simulink library "AEMS_Standard_Library"  (R2016b)
settings: Solver=ode45  StartTime=0.0  StopTime=10.0  RelTol=1e-3
undefined symbols (not defined in the file or in its folder): BkPY, carto, Cbx_extegr, Cbx_lpegrsys, Cbx_portegr, Cnx_bnk_nr_conf, Cnx_cyl_nr_conf, ConfigManagement, configuration_management, Cxx_dcm_io_tmr_end_xxxx, Cxx_dcm_rt_tmr_end, Cxx_DID_xxxx_IO_max, Cxx_DID_xxxx_IO_min, Cxx_egrhsofs, Cxx_vmaniegi, DEM_DEBOUNCE_FREEZE, DEM_DTR_CTL_INVISIBLE, DEM_DTR_CTL_NORMAL, Dem_DtrId2_XXX, Dem_DtrId3_XXX, Dem_DtrId4_XXX, Dem_DtrId5_XXX, Dem_DtrId6_XXX, Dem_DtrId7_XXX, Dem_DtrId8_XXX, Dem_DtrId9_XXX, Dem_DtrId_XXX, Dem_EnableConditionId2_XXX, Dem_EnableConditionId3_XXX, Dem_EnableConditionId4_XXX, Dem_EnableConditionId5_XXX, Dem_EnableConditionId6_XXX, Dem_EnableConditionId7_XXX, Dem_EnableConditionId8_XXX, Dem_EnableConditionId_XXX, Dem_EventId, Dem_EventId2_XXX, Dem_EventId3_XXX, Dem_EventId4_XXX, Dem_EventId5_XXX, Dem_EventId6_XXX, Dem_EventId7_XXX, Dem_EventId8_XXX, Dem_EventId9_XXX, Dem_EventId_Device_Faulttype, Dem_EventId_XXX, DEM_IUMPR_GENERAL_DENOMINATOR, DEM_OPCYC_IGNITION, Dem_RatioId2_XXX, Dem_RatioId3_XXX, Dem_RatioId4_XXX, Dem_RatioId5_XXX, Dem_RatioId6_XXX, Dem_RatioId7_XXX, Dem_RatioId8_XXX, Dem_RatioId_XXX, Dem_StorageConditionId2_XXX, Dem_StorageConditionId3_XXX, Dem_StorageConditionId4_XXX, Dem_StorageConditionId5_XXX ... (+65)
libraries: AEMS_Standard_Library x477, simulink x2
(part 36 of 39)

== system AEMS_Standard_Library/SUB/AEMS_SORT_MEDIAN/Pair ==
  Vector_size : Inport
  Sorted_vector : Inport  Port=2
  Action Port : ActionPort
  Add : Sum  OutDataTypeStr=Inherit: Inherit via back propagation
  Add1 : Sum  OutDataTypeStr=Inherit: Inherit via back propagation  SaturateOnIntegerOverflow=on  InputSameDT=on
  Constant : Constant  Value=2  OutDataTypeStr=uint8
  Constant1 : Constant  OutDataTypeStr=uint8
  Constant2 : Constant  Value=2  OutDataTypeStr=uint8
  Divide : Product  Inputs=*/  OutDataTypeStr=Inherit: Inherit via back propagation
  Divide1 : Product  Inputs=*/  OutDataTypeStr=Inherit: Inherit via back propagation
  Selector : Selector  IndexMode=Zero-based  InputPortWidth=N  IndexOptions=Index vector (port)  Indices=[1 3]  OutputSizes=1
  Selector1 : Selector  IndexMode=Zero-based  InputPortWidth=N  IndexOptions=Index vector (port)  Indices=[1 3]  OutputSizes=1
  Median_Pair : Outport
  wires:
  Constant/1 -> Divide/2
  Divide/1 -> Selector/2, Add/1
  Constant1/1 -> Add/2
  Add/1 -> Selector1/2
  Selector/1 -> Add1/1
  Selector1/1 -> Add1/2
  Add1/1 -> Divide1/1
  Constant2/1 -> Divide1/2
  Divide1/1 -> Median_Pair/1
  Vector_size/1 -> Divide/1
  Sorted_vector/1 -> Selector1/1, Selector/1

== system AEMS_Standard_Library/TIMER/AEMS_TIMER1/EdgeRising ==
  In : Inport
  DelayInput1 : UnitDelay  Description=\nStore in Global RAM  InitialCondition=initinit  SampleTime=-1
      settings: AttributesFormatString=IC = %<X0>
  LogicalOperator1 : Logic  OutDataTypeStr=boolean
  LogicalOperator3 : Logic  Operator=NOT  Inputs=1  OutDataTypeStr=boolean
  Out : Outport
  wires:
  LogicalOperator1/1 -> Out/1
  In/1 -> LogicalOperator1/1, DelayInput1/1
  DelayInput1/1 -> LogicalOperator3/1
  LogicalOperator3/1 -> LogicalOperator1/2

== system AEMS_Standard_Library/COM/AEMS_FRAME_SUPERVISION/ecu_frm_detection/C_mngt ==
  Frm_Detection_Cnd : Inport
  Status_Loc2 : Inport  Port=2
  Frm_Conf : Inport  Port=3
  Clear_Diag_Info_Counter : Inport  Port=4
  Frm_Detected_PREV : Inport  Port=5
  Constant10 : Constant  Value=0  OutDataTypeStr=Inherit: Inherit via back propagation
  Constant2 : Constant  OutDataTypeStr=Inherit: Inherit via back propagation
  Constant3 : Constant  Value=false
  Constant8 : Constant  Value=Nnx_pres_stt
  DataTypeConversion1 : DataTypeConversion  RndMeth=Zero
  LogicalOperator2 : Logic  Inputs=3  OutDataTypeStr=boolean
  LogicalOperator3 : Logic  Operator=OR  Inputs=3  OutDataTypeStr=boolean
  RelationalOperator1 : RelationalOperator  Operator===  OutDataTypeStr=boolean  RndMeth=Nearest  InputSameDT=on
  RelationalOperator2 : RelationalOperator  Operator===  OutDataTypeStr=boolean  RndMeth=Nearest  InputSameDT=on
  RelationalOperator7 : RelationalOperator  Operator===  OutDataTypeStr=boolean  RndMeth=Nearest  InputSameDT=on
  Switch : Switch  Criteria=u2 ~= 0
      settings: AttributesFormatString=Criteria=%<Criteria>
  Frm_Detected : Outport
  wires:
  Switch/1 -> DataTypeConversion1/1
  Clear_Diag_Info_Counter/1 -> Switch/2
  Constant10/1 -> RelationalOperator2/2
  RelationalOperator7/1 -> LogicalOperator2/3
  Constant8/1 -> RelationalOperator7/1
  Frm_Detection_Cnd/1 -> LogicalOperator2/2
  RelationalOperator2/1 -> LogicalOperator3/1
  LogicalOperator2/1 -> LogicalOperator3/2
  Frm_Conf/1 -> RelationalOperator2/1, RelationalOperator1/1
  RelationalOperator1/1 -> LogicalOperator2/1
  Constant2/1 -> RelationalOperator1/2
  Frm_Detected_PREV/1 -> LogicalOperator3/3
  LogicalOperator3/1 -> Switch/1
  DataTypeConversion1/1 -> Frm_Detected/1
  Status_Loc2/1 -> RelationalOperator7/2
  Constant3/1 -> Switch/3

== system AEMS_Standard_Library/COM/AEMS_FRAME_SUPERVISION/ecu_frm_monitoring/A_Monitoring_Condition ==
  GADE : Inport
  ECU_Category : Inport  Port=2
  IgnitionSupplyConfirmation : Inport  Port=3
  Specific_Mon_Cnd : Inport  Port=4
  Frame_Detected_Loc2 : Inport  Port=5
  BCM_Status : Inport  Port=6
  USM_Status : Inport  Port=7
  GADEOK : Constant  Value=3  OutDataTypeStr=Inherit: Inherit via back propagation
  LogicalOperator1 : Logic  OutDataTypeStr=boolean
  LogicalOperator2 : Logic  Inputs=3  OutDataTypeStr=boolean
  LogicalOperator3 : Logic  Operator=OR  OutDataTypeStr=boolean
  PRESENTSTATUS : Constant  Value=Nnx_pres_stt
  PRESENTSTATUS_102 : Constant  Value=Nnx_pres_stt
  RelationalOperator1 : RelationalOperator  Operator===  OutDataTypeStr=boolean  RndMeth=Nearest  InputSameDT=on
  RelationalOperator2 : RelationalOperator  Operator=~=  OutDataTypeStr=boolean  RndMeth=Nearest  InputSameDT=on
  RelationalOperator3 : RelationalOperator  Operator===  OutDataTypeStr=boolean  RndMeth=Nearest  InputSameDT=on
  Switch : Switch  Criteria=u2 ~= 0  RndMeth=Zero  InputSameDT=on
      settings: AttributesFormatString=Criteria=%<Criteria>
  Mon_Authorize : Outport
  wires:
  LogicalOperator3/1 -> Switch/1
  LogicalOperator1/1 -> Switch/3
  LogicalOperator2/1 -> Mon_Authorize/1
  BCM_Status/1 -> RelationalOperator1/1
  Frame_Detected_Loc2/1 -> LogicalOperator2/3
  Specific_Mon_Cnd/1 -> LogicalOperator2/2
  Switch/1 -> LogicalOperator2/1
  PRESENTSTATUS_102/1 -> RelationalOperator2/2
  USM_Status/1 -> RelationalOperator2/1
  PRESENTSTATUS/1 -> RelationalOperator1/2
  RelationalOperator2/1 -> LogicalOperator3/2
  IgnitionSupplyConfirmation/1 -> LogicalOperator3/1
  RelationalOperator1/1 -> LogicalOperator1/1
  RelationalOperator3/1 -> LogicalOperator1/2
  GADEOK/1 -> RelationalOperator3/2
  GADE/1 -> RelationalOperator3/1
  ECU_Category/1 -> Switch/2

== system AEMS_Standard_Library/COM/AEMS_FRAME_SUPERVISION/ecu_frm_monitoring/B_Status_Management ==
  rcpt_frm : Inport
  Mon_Authorize : Inport  Port=2
  TimeSched_dt : Inport  Port=3
  JT1 : Inport  Port=4
  JT2 : Inport  Port=5
  Vbx_atsr_sys_ecu_ini_task10ms : Inport  Port=6
  Frame_Detected : Inport  Port=7
  C_Status_building : Subsystem
  Constant : Constant  Value=Nnx_pres_stt
  Constant1 : Constant  Value=Nnx_abst_stt
  Switch : Switch  Criteria=u2 ~= 0
      settings: AttributesFormatString=Criteria=%<Criteria>
  Switch3 : Switch  Criteria=u2 ~= 0  RndMeth=Zero  InputSameDT=on
      settings: AttributesFormatString=Criteria=%<Criteria>
  Unit Delay : UnitDelay  SampleTime=-1
      settings: AttributesFormatString=<initial=%<InitialCondition>>
  Status : Outport
  wires:
  Unit Delay/1 -> C_Status_building/6(Status_PREV)
  Switch/1 -> Status/1, Unit Delay/1
  rcpt_frm/1 -> C_Status_building/5(Frame_Received)
  Frame_Detected/1 -> Switch3/2
  Constant/1 -> Switch3/1
  Constant1/1 -> Switch3/3
  Vbx_atsr_sys_ecu_ini_task10ms/1 -> Switch/2
  Mon_Authorize/1 -> C_Status_building/1(Mon_Authorize)
  TimeSched_dt/1 -> C_Status_building/2(TimeSched_dt)
  JT1/1 -> C_Status_building/3(JT1)
  JT2/1 -> C_Status_building/4(JT2)
  Switch3/1 -> Switch/1
  C_Status_building/1(Status) -> Switch/3

== system AEMS_Standard_Library/COM/AEMS_FRAME_SUPERVISION/ecu_monitoring_display/D_ctr_mem_max ==
  VALMAX : Inport
  M_Absent_PREV : Inport  Port=2
  Vbx_rcpt_XXX_mon_PREV : Inport  Port=3
  IGN_Status : Inport  Port=4
  decM : Inport  Port=5
  decThres : Inport  Port=6
  Frame_Received_Counter : Inport  Port=7
  Clear_Diag_Info_Counter : Inport  Port=8
  Status : Inport  Port=9
  Constant : Constant  Value=Nnx_vld_abst_stt
  Constant1 : Constant  Value=0  OutDataTypeStr=Inherit: Inherit via back propagation
  Constant2 : Constant  Value=0  OutDataTypeStr=Inherit: Inherit via back propagation
  DataTypeConversion2 : DataTypeConversion  RndMeth=Zero
  LogicalOperator : Logic  Operator=NOT  OutDataTypeStr=boolean
  LogicalOperator1 : Logic  Operator=OR  OutDataTypeStr=boolean
  LogicalOperator2 : Logic  Operator=OR  OutDataTypeStr=boolean
  LogicalOperator3 : Logic  Inputs=3  OutDataTypeStr=boolean
  MinMax : MinMax  Function=max  Inputs=2  OutDataTypeStr=Inherit: Inherit via back propagation  RndMeth=Zero  InputSameDT=on
  RelationalOperator2 : RelationalOperator  Operator=~=  OutDataTypeStr=boolean  RndMeth=Nearest  InputSameDT=on
  RelationalOperator4 : RelationalOperator  Operator===  OutDataTypeStr=boolean  RndMeth=Nearest  InputSameDT=on
  RelationalOperator5 : RelationalOperator  Operator=<  OutDataTypeStr=boolean  RndMeth=Nearest  InputSameDT=on
  Subtract : Sum  Inputs=+-  OutDataTypeStr=Inherit: Inherit via back propagation  RndMeth=Zero  InputSameDT=on
  Switch{1..6} (6 alike) : Switch  Criteria=u2 ~= 0  RndMeth=Zero  SaturateOnIntegerOverflow=on  InputSameDT=on
      settings: AttributesFormatString=Criteria=%<Criteria>
  M_Absent : Outport
  Vbx_rcpt_XXX_mon : Outport  Port=2
  wires:
  Frame_Received_Counter/1 -> Switch5/2, Switch6/2
  Constant/1 -> RelationalOperator4/2
  Status/1 -> RelationalOperator4/1
  VALMAX/1 -> Switch1/1
  RelationalOperator4/1 -> LogicalOperator1/1, Switch1/2
  Switch6/1 -> Vbx_rcpt_XXX_mon/1
  LogicalOperator1/1 -> Switch6/1
  LogicalOperator2/1 -> Switch6/3
  Switch1/1 -> Switch5/1
  LogicalOperator3/1 -> Switch4/2
  Vbx_rcpt_XXX_mon_PREV/1 -> LogicalOperator1/2, LogicalOperator/1, LogicalOperator2/1
  Constant1/1 -> RelationalOperator2/2
  M_Absent_PREV/1 -> Subtract/1, Switch4/3, RelationalOperator2/1, Switch2/3, RelationalOperator5/2, Switch1/3
  RelationalOperator2/1 -> LogicalOperator3/3
  IGN_Status/1 -> LogicalOperator2/2, LogicalOperator3/2
  LogicalOperator/1 -> LogicalOperator3/1
  Switch4/1 -> Switch5/3
  Switch5/1 -> Switch3/1
  Switch3/1 -> DataTypeConversion2/1
  Clear_Diag_Info_Counter/1 -> Switch3/2
  Constant2/1 -> Switch3/3
  DataTypeConversion2/1 -> M_Absent/1
  RelationalOperator5/1 -> Switch2/2
  decM/1 -> Switch2/1, RelationalOperator5/1
  Switch2/1 -> Subtract/2
  Subtract/1 -> MinMax/1
  decThres/1 -> MinMax/2
  MinMax/1 -> Switch4/1

== system AEMS_Standard_Library/COM/AEMS_FRAME_SUPERVISION/ecu_monitoring_display/E_diag_display ==
  note: b1000 0000
  note: b1100 0000
  note: b1111 1111
  note: b0011 1111
  M_Absent : Inport
  Mon_Authorized : Inport  Port=2
  Dspl_Mask_Cnd : Inport  Port=3
  Status : Inport  Port=4
  Constant : Constant  Value=Nnx_vld_abst_stt
  Constant1 : Constant  Value=Nnx_abst_stt
  Constant10 : Constant  Value=0  OutDataTypeStr=Inherit: Inherit via back propagation
  Constant2 : Constant  Value=63  OutDataTypeStr=Inherit: Inherit via back propagation
  Constant6 : Constant  Value=255  OutDataTypeStr=Inherit: Inherit via back propagation
  Constant7 : Constant  Value=128  OutDataTypeStr=Inherit: Inherit via back propagation
  Constant8 : Constant  Value=0  OutDataTypeStr=Inherit: Inherit via back propagation
  Constant9 : Constant  Value=192  OutDataTypeStr=Inherit: Inherit via back propagation
  LogicalOperator1 : Logic  Operator=NOT  Inputs=1  OutDataTypeStr=boolean
  LogicalOperator8 : Logic  Operator=OR  OutDataTypeStr=boolean
  MinMax : MinMax  Inputs=2  OutDataTypeStr=Inherit: Inherit via back propagation  RndMeth=Zero  InputSameDT=on
  RelationalOperator3 : RelationalOperator  Operator===  OutDataTypeStr=boolean  RndMeth=Nearest  InputSameDT=on
  RelationalOperator4 : RelationalOperator  Operator===  OutDataTypeStr=boolean  RndMeth=Nearest  InputSameDT=on
  Sum : Sum  Inputs=2  OutDataTypeStr=Inherit: Inherit via back propagation  RndMeth=Zero  InputSameDT=on
  Sum1 : Sum  Inputs=2  OutDataTypeStr=Inherit: Inherit via back propagation  RndMeth=Zero  InputSameDT=on
  Switch1 : Switch  Criteria=u2 ~= 0  RndMeth=Zero  SaturateOnIntegerOverflow=on  InputSameDT=on
      settings: AttributesFormatString=Criteria=%<Criteria>
  Switch2 : Switch  Criteria=u2 ~= 0  RndMeth=Zero  SaturateOnIntegerOverflow=on  InputSameDT=on
      settings: AttributesFormatString=Criteria=%<Criteria>
  Switch3 : Switch  Criteria=u2 ~= 0  RndMeth=Zero  SaturateOnIntegerOverflow=on  InputSameDT=on
      settings: AttributesFormatString=Criteria=%<Criteria>
  Diagnosis_Byte : Outport
  wires:
  LogicalOperator8/1 -> Switch1/2
  Constant6/1 -> Switch1/1
  Status/1 -> RelationalOperator3/1, RelationalOperator4/2
  Constant/1 -> RelationalOperator3/2
  Constant1/1 -> RelationalOperator4/1
  RelationalOperator4/1 -> Switch2/2
  Constant7/1 -> Switch2/1
  Constant8/1 -> Switch2/3
  RelationalOperator3/1 -> Switch3/2
  Constant9/1 -> Switch3/1
  Constant10/1 -> Switch3/3
  Switch1/1 -> Diagnosis_Byte/1
  Mon_Authorized/1 -> LogicalOperator1/1
  LogicalOperator1/1 -> LogicalOperator8/1
  Dspl_Mask_Cnd/1 -> LogicalOperator8/2
  M_Absent/1 -> MinMax/1
  Constant2/1 -> MinMax/2
  Sum1/1 -> Switch1/3
  MinMax/1 -> Sum/1
  Switch2/1 -> Sum/2
  Switch3/1 -> Sum1/2
  Sum/1 -> Sum1/1

== system AEMS_Standard_Library/DCM/AEMS_DCM_CLEARDIAGNOSTICINFORMATION/Callback_Subsystem/Enable_Clear_Request_Subsystem ==
  Enable : EnablePort
  Logical Operator3 : Logic  Operator=NOT  OutDataTypeStr=boolean
  Unit Delay1 : UnitDelay  SampleTime=-1
      settings: AttributesFormatString=<initial=%<InitialCondition>>
  flag_clr_req : Outport  InitialOutput=0
      settings: AttributesFormatString=<initial=%<InitialOutput>>\n<whendisabled=%<OutputWhenDisabled>>
  wires:
  Unit Delay1/1 -> Logical Operator3/1
  Logical Operator3/1 -> flag_clr_req/1, Unit Delay1/1

== system AEMS_Standard_Library/DISCONTINUITIES/AEMS_MULTI_PORT_TIME_SWITCH/slop_on/SR_FlipFlop1 ==
  S : Inport
  R : Inport  Port=2
  Constant1 : Constant  Value=false
  Constant2 : Constant  Value=true
  Constant3 : Constant  Value=true
  Constant5 : Constant  Value=false
  Logical_Operator : Logic  OutDataTypeStr=boolean
  Logical_Operator3 : Logic  Operator=NOT  OutDataTypeStr=boolean
  Relational_Operator : RelationalOperator  Operator===  OutDataTypeStr=boolean  RndMeth=Nearest  InputSameDT=on
  Switch{,1..3} (4 alike) : Switch  Criteria=u2 ~= 0  RndMeth=Zero  InputSameDT=on
      settings: AttributesFormatString=Criteria=%<Criteria>
  Unit_Delay : UnitDelay  SampleTime=-1
      settings: AttributesFormatString=IC = %<X0>
  Q : Outport
  QNot : Outport  Port=2
  wires:
  Logical_Operator3/1 -> QNot/1
  S/1 -> Switch/2, Logical_Operator/2
  R/1 -> Switch1/2, Logical_Operator/1
  Constant3/1 -> Switch/1
  Switch1/1 -> Switch/3
  Constant5/1 -> Switch1/1
  Unit_Delay/1 -> Relational_Operator/1, Switch1/3
  Switch3/1 -> Logical_Operator3/1, Q/1, Unit_Delay/1
  Logical_Operator/1 -> Switch3/2, Relational_Operator/2
  Relational_Operator/1 -> Switch2/2
  Constant2/1 -> Switch2/1
  Constant1/1 -> Switch2/3
  Switch2/1 -> Switch3/1
  Switch/1 -> Switch3/3

== system AEMS_Standard_Library/DISCONTINUITIES/AEMS_MULTI_PORT_TIME_SWITCH/transient_timer/AEMS_DIVISION_BY_ZERO ==
  den : Inport  Tag=AM,In,0,1,Name,C;CMP,Port,PortWidth,SampleTime;
  num : Inport  Tag=AM,In,0,1,Name,C;CMP,Port,PortWidth,SampleTime;  Port=2
  ans_of_0div : Inport  Tag=AM,In,0,1,Name,C;CMP,Port,PortWidth,SampleTime;  Port=3
  Divide : Product  Inputs=*/  OutDataTypeStr=Inherit: Inherit via back propagation  RndMeth=Zero
  MinMax1 : MinMax  Function=max  Inputs=2  OutDataTypeStr=Inherit: Inherit via back propagation  RndMeth=Zero  InputSameDT=on
  RelationalOperator : RelationalOperator  Tag=AM,Std,2,1;CMP,Operator;  Operator=~=  OutDataTypeStr=boolean  RndMeth=Nearest  InputSameDT=on
  Switch2 : Switch  Tag=GEN,Threshold;AM,Switch,2,1;CMP,Threshold;  Criteria=u2 ~= 0  RndMeth=Zero  SaturateOnIntegerOverflow=on  InputSameDT=on
      settings: AttributesFormatString=Criteria=%<Criteria>
  imm_zero : Constant  Tag=AM,Constant,0,1,Value;CMP,Value;  Value=0  OutDataTypeStr=Inherit: Inherit via back propagation
  imm_zero3 : Constant  Tag=AM,Constant,0,1,Value;CMP,Value;  Value=0.064/2^53  OutDataTypeStr=Inherit: Inherit via back propagation
  ans : Outport  Tag=AM,Out,1,0,Name,NC;CMP,Port,OutputWhenDisabled,InitialOutput;
  wires:
  den/1 -> RelationalOperator/1, MinMax1/1
  imm_zero/1 -> RelationalOperator/2
  num/1 -> Divide/1
  imm_zero3/1 -> MinMax1/2
  RelationalOperator/1 -> Switch2/2
  ans_of_0div/1 -> Switch2/3
  MinMax1/1 -> Divide/2
  Divide/1 -> Switch2/1
  Switch2/1 -> ans/1

== system AEMS_Standard_Library/DISCONTINUITIES/AEMS_SLEW_RATE/Slew_rate/Slewing ==
  OUTPUT_Prev : Inport
  MAX_SLEW_RATE : Inport  Port=2
  MIN_SLEW_RATE : Inport  Port=3
  INPUT : Inport  Port=4
  RelationalOperator : RelationalOperator  Operator=<=  OutDataTypeStr=boolean  RndMeth=Nearest  InputSameDT=on
  RelationalOperator1 : RelationalOperator  OutDataTypeStr=boolean  RndMeth=Nearest  InputSameDT=on
  Sum : Sum  Inputs=+-  OutDataTypeStr=Inherit: Inherit via back propagation  RndMeth=Zero  InputSameDT=on
  Sum1 : Sum  OutDataTypeStr=Inherit: Inherit via back propagation  RndMeth=Zero  InputSameDT=on
  Switch : Switch  Criteria=u2 ~= 0  RndMeth=Zero  SaturateOnIntegerOverflow=on  InputSameDT=on
      settings: AttributesFormatString=Criteria=%<Criteria>
  Switch1 : Switch  Criteria=u2 ~= 0  RndMeth=Zero  SaturateOnIntegerOverflow=on  InputSameDT=on
      settings: AttributesFormatString=Criteria=%<Criteria>
  OUTPUT : Outport  InitialOutput=0
  wires:
  Sum1/1 -> OUTPUT/1
  INPUT/1 -> Sum/1
  MIN_SLEW_RATE/1 -> RelationalOperator1/2, Switch1/3
  Switch/1 -> Sum1/2
  OUTPUT_Prev/1 -> Sum1/1, Sum/2
  RelationalOperator/1 -> Switch/2
  Sum/1 -> RelationalOperator/2, RelationalOperator1/1, Switch1/1
  RelationalOperator1/1 -> Switch1/2
  Switch1/1 -> Switch/3
  MAX_SLEW_RATE/1 -> RelationalOperator/1, Switch/1

== system AEMS_Standard_Library/DISCONTINUITIES/AEMS_SLOPE_SWITCH/Slope_On_Block/Error_Due_To_High_Slope_Test ==
  Signal_Change : Inport
  Output_Less_Than_Input : Inport  Port=2
  Output_Greater_Than_Input : Inport  Port=3
  Logical_Operator1 : Logic  Operator=OR  OutDataTypeStr=boolean
  Relational_Operator3 : RelationalOperator  Operator=~=  OutDataTypeStr=boolean  RndMeth=Nearest  InputSameDT=on
  Unit_Delay1 : UnitDelay  SampleTime=-1
      settings: AttributesFormatString=IC = %<X0>
  Test_passed : Outport
  wires:
  Logical_Operator1/1 -> Test_passed/1
  Signal_Change/1 -> Logical_Operator1/1
  Output_Less_Than_Input/1 -> Unit_Delay1/1
  Output_Greater_Than_Input/1 -> Relational_Operator3/1
  Relational_Operator3/1 -> Logical_Operator1/2
  Unit_Delay1/1 -> Relational_Operator3/2

== system AEMS_Standard_Library/DISCONTINUITIES/AEMS_SLOPE_SWITCH/Slope_On_Block/Output_Comparision ==
  Test_passed : Inport
  Input : Inport  Tag=AM,In,0,1,Name,C;CMP,Port,PortWidth,SampleTime;  Port=2
  Pos_Slope : Inport  Tag=AM,In,0,1,Name,C;CMP,Port,PortWidth,SampleTime;  Port=3
  Prev_Output : Inport  Port=4
  Neg_Slope : Inport  Tag=AM,In,0,1,Name,C;CMP,Port,PortWidth,SampleTime;  Port=5
  Logical_Operator : Logic  Operator=OR  OutDataTypeStr=boolean
  Logical_Operator2 : Logic  OutDataTypeStr=boolean
  Relational_Operator1 : RelationalOperator  Operator=>  OutDataTypeStr=boolean  RndMeth=Nearest  InputSameDT=on
  Relational_Operator2 : RelationalOperator  Operator=<  OutDataTypeStr=boolean  RndMeth=Nearest  InputSameDT=on
  Sum : Sum  OutDataTypeStr=Inherit: Inherit via back propagation  RndMeth=Zero  SaturateOnIntegerOverflow=on  InputSameDT=on
      settings: AttributesFormatString=SAT = %<SaturateOnIntegerOverflow>
  Sum1 : Sum  OutDataTypeStr=Inherit: Inherit via back propagation  RndMeth=Zero  SaturateOnIntegerOverflow=on  InputSameDT=on
      settings: AttributesFormatString=SAT = %<SaturateOnIntegerOverflow>
  Switch1 : Switch  Tag=GEN,Threshold;AM,Switch,2,1;CMP,Threshold;  Criteria=u2 ~= 0  RndMeth=Zero  SaturateOnIntegerOverflow=on  InputSameDT=on
      settings: AttributesFormatString=Criteria=%<Criteria>
  Switch2 : Switch  Tag=GEN,Threshold;AM,Switch,2,1;CMP,Threshold;  Criteria=u2 ~= 0  RndMeth=Zero  SaturateOnIntegerOverflow=on  InputSameDT=on
      settings: AttributesFormatString=Criteria=%<Criteria>
  Switch3 : Switch  Tag=GEN,Threshold;AM,Switch,2,1;CMP,Threshold;  Criteria=u2 ~= 0  RndMeth=Zero  SaturateOnIntegerOverflow=on  InputSameDT=on
      settings: AttributesFormatString=Criteria=%<Criteria>
  Output_Not_Equals_Input : Outport  Tag=AM,Out,1,0,Name,NC;CMP,Port,OutputWhenDisabled,InitialOutput;
  Output : Outport  Tag=AM,Out,1,0,Name,NC;CMP,Port,OutputWhenDisabled,InitialOutput;  Port=2
  RelOp2_out : Outport  Tag=AM,Out,1,0,Name,NC;CMP,Port,OutputWhenDisabled,InitialOutput;  Port=3
  RelOp1_out : Outport  Tag=AM,Out,1,0,Name,NC;CMP,Port,OutputWhenDisabled,InitialOutput;  Port=4
  wires:
  Relational_Operator1/1 -> RelOp1_out/1, Switch1/2, Logical_Operator/2
  Relational_Operator2/1 -> RelOp2_out/1, Switch2/2, Logical_Operator/1
  Sum/1 -> Switch1/1, Relational_Operator1/1
  Input/1 -> Switch1/3, Relational_Operator2/2, Switch3/3, Relational_Operator1/2
  Switch2/1 -> Switch3/1
  Switch1/1 -> Switch2/3
  Prev_Output/1 -> Sum1/1, Sum/1
  Logical_Operator2/1 -> Output_Not_Equals_Input/1
  Logical_Operator/1 -> Logical_Operator2/2
  Switch3/1 -> Output/1
  Test_passed/1 -> Switch3/2, Logical_Operator2/1
  Sum1/1 -> Relational_Operator2/1, Switch2/1
  Pos_Slope/1 -> Sum1/2
  Neg_Slope/1 -> Sum/2

== system AEMS_Standard_Library/DISCONTINUITIES/AEMS_SLOPE_SWITCH_3INPUTS/Slope_On_Block/Error_Due_To_High_Slope_Test ==
  Signal_Change : Inport
  Output_Greater_Than_Input : Inport  Port=2
  Output_Less_Than_Input : Inport  Port=3
  Logical_Operator1 : Logic  Operator=OR  OutDataTypeStr=boolean
  Relational_Operator3 : RelationalOperator  Operator=~=  OutDataTypeStr=boolean  RndMeth=Nearest  InputSameDT=on
  Unit_Delay1 : UnitDelay  SampleTime=-1
      settings: AttributesFormatString=IC = %<X0>
  Test_passed : Outport
  wires:
  Unit_Delay1/1 -> Relational_Operator3/2
  Relational_Operator3/1 -> Logical_Operator1/2
  Output_Greater_Than_Input/1 -> Relational_Operator3/1
  Output_Less_Than_Input/1 -> Unit_Delay1/1
  Signal_Change/1 -> Logical_Operator1/1
  Logical_Operator1/1 -> Test_passed/1

== system AEMS_Standard_Library/DISCONTINUITIES/AEMS_SLOPE_SWITCH_3INPUTS/Slope_On_Block/Output_Comparision ==
  Test_passed : Inport
  Input : Inport  Tag=AM,In,0,1,Name,C;CMP,Port,PortWidth,SampleTime;  Port=2
  Pos_Slope : Inport  Tag=AM,In,0,1,Name,C;CMP,Port,PortWidth,SampleTime;  Port=3
  Prev_Output : Inport  Port=4
  Neg_Slope : Inport  Tag=AM,In,0,1,Name,C;CMP,Port,PortWidth,SampleTime;  Port=5
  LogicalOperator : Logic  Operator=OR  OutDataTypeStr=boolean
  Logical_Operator2 : Logic  OutDataTypeStr=boolean
  Relational_Operator1 : RelationalOperator  Operator=>  OutDataTypeStr=boolean  RndMeth=Nearest  InputSameDT=on
  Relational_Operator2 : RelationalOperator  Operator=<  OutDataTypeStr=boolean  RndMeth=Nearest  InputSameDT=on
  Sum : Sum  OutDataTypeStr=Inherit: Inherit via back propagation  RndMeth=Zero  SaturateOnIntegerOverflow=on  InputSameDT=on
      settings: AttributesFormatString=SAT = %<SaturateOnIntegerOverflow>
  Sum1 : Sum  OutDataTypeStr=Inherit: Inherit via back propagation  RndMeth=Zero  SaturateOnIntegerOverflow=on  InputSameDT=on
      settings: AttributesFormatString=SAT = %<SaturateOnIntegerOverflow>
  Switch1 : Switch  Tag=GEN,Threshold;AM,Switch,2,1;CMP,Threshold;  Criteria=u2 ~= 0  RndMeth=Zero  SaturateOnIntegerOverflow=on  InputSameDT=on
      settings: AttributesFormatString=Criteria=%<Criteria>
  Switch2 : Switch  Tag=GEN,Threshold;AM,Switch,2,1;CMP,Threshold;  Criteria=u2 ~= 0  RndMeth=Zero  SaturateOnIntegerOverflow=on  InputSameDT=on
      settings: AttributesFormatString=Criteria=%<Criteria>
  Switch3 : Switch  Tag=GEN,Threshold;AM,Switch,2,1;CMP,Threshold;  Criteria=u2 ~= 0  RndMeth=Zero  SaturateOnIntegerOverflow=on  InputSameDT=on
      settings: AttributesFormatString=Criteria=%<Criteria>
  Output_Not_Equals_Input : Outport  Tag=AM,Out,1,0,Name,NC;CMP,Port,OutputWhenDisabled,InitialOutput;
  Output : Outport  Tag=AM,Out,1,0,Name,NC;CMP,Port,OutputWhenDisabled,InitialOutput;  Port=2
  RelOp2_out : Outport  Tag=AM,Out,1,0,Name,NC;CMP,Port,OutputWhenDisabled,InitialOutput;  Port=3
  RelOp1_out : Outport  Tag=AM,Out,1,0,Name,NC;CMP,Port,OutputWhenDisabled,InitialOutput;  Port=4
  wires:
  Prev_Output/1 -> Sum1/1, Sum/1
  Neg_Slope/1 -> Sum/2
  Pos_Slope/1 -> Sum1/2
  Sum1/1 -> Switch2/1, Relational_Operator2/1
  Test_passed/1 -> Logical_Operator2/1, Switch3/2
  Switch3/1 -> Output/1
  LogicalOperator/1 -> Logical_Operator2/2
  Logical_Operator2/1 -> Output_Not_Equals_Input/1
  Switch1/1 -> Switch2/3
  Switch2/1 -> Switch3/1
  Input/1 -> Switch1/3, Relational_Operator1/2, Relational_Operator2/2, Switch3/3
  Sum/1 -> Relational_Operator1/1, Switch1/1
  Relational_Operator2/1 -> LogicalOperator/1, RelOp2_out/1, Switch2/2
  Relational_Operator1/1 -> LogicalOperator/2, Switch1/2, RelOp1_out/1

== system AEMS_Standard_Library/DISCONTINUITIES/AEMS_SLOPE_SWITCH_4INPUTS/Slope_On_Block/Error_Due_To_High_Slope_Test ==
  Signal_Change : Inport
  Output_Greater_Than_Input : Inport  Port=2
  Output_Less_Than_Input : Inport  Port=3
  Logical_Operator1 : Logic  Operator=OR  OutDataTypeStr=boolean
  Relational_Operator3 : RelationalOperator  Operator=~=  OutDataTypeStr=boolean  RndMeth=Nearest  InputSameDT=on
  Unit_Delay1 : UnitDelay  SampleTime=-1
      settings: AttributesFormatString=IC = %<X0>
  Test_passed : Outport
  wires:
  Unit_Delay1/1 -> Relational_Operator3/2
  Relational_Operator3/1 -> Logical_Operator1/2
  Output_Greater_Than_Input/1 -> Relational_Operator3/1
  Output_Less_Than_Input/1 -> Unit_Delay1/1
  Signal_Change/1 -> Logical_Operator1/1
  Logical_Operator1/1 -> Test_passed/1

== system AEMS_Standard_Library/DISCONTINUITIES/AEMS_SLOPE_SWITCH_4INPUTS/Slope_On_Block/Output_Comparision ==
  Test_passed : Inport
  Input : Inport  Tag=AM,In,0,1,Name,C;CMP,Port,PortWidth,SampleTime;  Port=2
  Pos_Slope : Inport  Tag=AM,In,0,1,Name,C;CMP,Port,PortWidth,SampleTime;  Port=3
  Prev_Output : Inport  Port=4
  Neg_Slope : Inport  Tag=AM,In,0,1,Name,C;CMP,Port,PortWidth,SampleTime;  Port=5
  LogicalOperator : Logic  Operator=OR  OutDataTypeStr=boolean
  Logical_Operator2 : Logic  OutDataTypeStr=boolean
  Relational_Operator1 : RelationalOperator  Operator=>  OutDataTypeStr=boolean  RndMeth=Nearest  InputSameDT=on
  Relational_Operator2 : RelationalOperator  Operator=<  OutDataTypeStr=boolean  RndMeth=Nearest  InputSameDT=on
  Sum : Sum  OutDataTypeStr=Inherit: Inherit via back propagation  RndMeth=Zero  SaturateOnIntegerOverflow=on  InputSameDT=on
      settings: AttributesFormatString=SAT = %<SaturateOnIntegerOverflow>
  Sum1 : Sum  OutDataTypeStr=Inherit: Inherit via back propagation  RndMeth=Zero  SaturateOnIntegerOverflow=on  InputSameDT=on
      settings: AttributesFormatString=SAT = %<SaturateOnIntegerOverflow>
  Switch1 : Switch  Tag=GEN,Threshold;AM,Switch,2,1;CMP,Threshold;  Criteria=u2 ~= 0  RndMeth=Zero  SaturateOnIntegerOverflow=on  InputSameDT=on
      settings: AttributesFormatString=Criteria=%<Criteria>
  Switch2 : Switch  Tag=GEN,Threshold;AM,Switch,2,1;CMP,Threshold;  Criteria=u2 ~= 0  RndMeth=Zero  SaturateOnIntegerOverflow=on  InputSameDT=on
      settings: AttributesFormatString=Criteria=%<Criteria>
  Switch3 : Switch  Tag=GEN,Threshold;AM,Switch,2,1;CMP,Threshold;  Criteria=u2 ~= 0  RndMeth=Zero  SaturateOnIntegerOverflow=on  InputSameDT=on
      settings: AttributesFormatString=Criteria=%<Criteria>
  Output_Not_Equals_Input : Outport  Tag=AM,Out,1,0,Name,NC;CMP,Port,OutputWhenDisabled,InitialOutput;
  Output : Outport  Tag=AM,Out,1,0,Name,NC;CMP,Port,OutputWhenDisabled,InitialOutput;  Port=2
  RelOp2_out : Outport  Tag=AM,Out,1,0,Name,NC;CMP,Port,OutputWhenDisabled,InitialOutput;  Port=3
  RelOp1_out : Outport  Tag=AM,Out,1,0,Name,NC;CMP,Port,OutputWhenDisabled,InitialOutput;  Port=4
  wires:
  Prev_Output/1 -> Sum1/1, Sum/1
  Neg_Slope/1 -> Sum/2
  Pos_Slope/1 -> Sum1/2
  Sum1/1 -> Switch2/1, Relational_Operator2/1
  Test_passed/1 -> Logical_Operator2/1, Switch3/2
  Switch3/1 -> Output/1
  LogicalOperator/1 -> Logical_Operator2/2
  Logical_Operator2/1 -> Output_Not_Equals_Input/1
  Switch1/1 -> Switch2/3
  Switch2/1 -> Switch3/1
  Input/1 -> Switch1/3, Relational_Operator1/2, Relational_Operator2/2, Switch3/3
  Sum/1 -> Relational_Operator1/1, Switch1/1
  Relational_Operator2/1 -> LogicalOperator/1, RelOp2_out/1, Switch2/2
  Relational_Operator1/1 -> LogicalOperator/2, Switch1/2, RelOp1_out/1

== system AEMS_Standard_Library/DISCONTINUITIES/AEMS_SLOPE_SWITCH_6INPUTS/Slope_On_Block/Error_Due_To_High_Slope_Test ==
  Signal_Change : Inport
  Output_Less_Than_Input : Inport  Port=2
  Output_Greater_Than_Input : Inport  Port=3
  Logical_Operator1 : Logic  Operator=OR  OutDataTypeStr=boolean
  Relational_Operator3 : RelationalOperator  Operator=~=  OutDataTypeStr=boolean  RndMeth=Nearest  InputSameDT=on
  Unit_Delay1 : UnitDelay  SampleTime=-1
      settings: AttributesFormatString=IC = %<X0>
  Test_passed : Outport
  wires:
  Logical_Operator1/1 -> Test_passed/1
  Signal_Change/1 -> Logical_Operator1/1
  Output_Less_Than_Input/1 -> Unit_Delay1/1
  Output_Greater_Than_Input/1 -> Relational_Operator3/1
  Relational_Operator3/1 -> Logical_Operator1/2
  Unit_Delay1/1 -> Relational_Operator3/2

== system AEMS_Standard_Library/DISCONTINUITIES/AEMS_SLOPE_SWITCH_6INPUTS/Slope_On_Block/Output_Comparision ==
  Test_passed : Inport
  Input : Inport  Tag=AM,In,0,1,Name,C;CMP,Port,PortWidth,SampleTime;  Port=2
  Pos_Slope : Inport  Tag=AM,In,0,1,Name,C;CMP,Port,PortWidth,SampleTime;  Port=3
  Prev_Output : Inport  Port=4
  Neg_Slope : Inport  Tag=AM,In,0,1,Name,C;CMP,Port,PortWidth,SampleTime;  Port=5
  LogicalOperator : Logic  Operator=OR  OutDataTypeStr=boolean
  Logical_Operator2 : Logic  OutDataTypeStr=boolean
  Relational_Operator1 : RelationalOperator  Operator=>  OutDataTypeStr=boolean  RndMeth=Nearest  InputSameDT=on
  Relational_Operator2 : RelationalOperator  Operator=<  OutDataTypeStr=boolean  RndMeth=Nearest  InputSameDT=on
  Sum : Sum  OutDataTypeStr=Inherit: Inherit via back propagation  RndMeth=Zero  SaturateOnIntegerOverflow=on  InputSameDT=on
      settings: AttributesFormatString=SAT = %<SaturateOnIntegerOverflow>
  Sum1 : Sum  OutDataTypeStr=Inherit: Inherit via back propagation  RndMeth=Zero  SaturateOnIntegerOverflow=on  InputSameDT=on
      settings: AttributesFormatString=SAT = %<SaturateOnIntegerOverflow>
  Switch1 : Switch  Tag=GEN,Threshold;AM,Switch,2,1;CMP,Threshold;  Criteria=u2 ~= 0  RndMeth=Zero  SaturateOnIntegerOverflow=on  InputSameDT=on
      settings: AttributesFormatString=Criteria=%<Criteria>
  Switch2 : Switch  Tag=GEN,Threshold;AM,Switch,2,1;CMP,Threshold;  Criteria=u2 ~= 0  RndMeth=Zero  SaturateOnIntegerOverflow=on  InputSameDT=on
      settings: AttributesFormatString=Criteria=%<Criteria>
  Switch3 : Switch  Tag=GEN,Threshold;AM,Switch,2,1;CMP,Threshold;  Criteria=u2 ~= 0  RndMeth=Zero  SaturateOnIntegerOverflow=on  InputSameDT=on
      settings: AttributesFormatString=Criteria=%<Criteria>
  Output_Not_Equals_Input : Outport  Tag=AM,Out,1,0,Name,NC;CMP,Port,OutputWhenDisabled,InitialOutput;
  Output : Outport  Tag=AM,Out,1,0,Name,NC;CMP,Port,OutputWhenDisabled,InitialOutput;  Port=2
  RelOp2_out : Outport  Tag=AM,Out,1,0,Name,NC;CMP,Port,OutputWhenDisabled,InitialOutput;  Port=3
  RelOp1_out : Outport  Tag=AM,Out,1,0,Name,NC;CMP,Port,OutputWhenDisabled,InitialOutput;  Port=4
  wires:
  Switch1/1 -> Switch2/3
  Relational_Operator2/1 -> RelOp2_out/1, LogicalOperator/1, Switch2/2
  Relational_Operator1/1 -> Switch1/2, LogicalOperator/2, RelOp1_out/1
  Sum/1 -> Relational_Operator1/1, Switch1/1
  Input/1 -> Relational_Operator2/2, Switch3/3, Relational_Operator1/2, Switch1/3
  Switch2/1 -> Switch3/1
  Logical_Operator2/1 -> Output_Not_Equals_Input/1
  LogicalOperator/1 -> Logical_Operator2/2
  Switch3/1 -> Output/1
  Test_passed/1 -> Switch3/2, Logical_Operator2/1
  Sum1/1 -> Relational_Operator2/1, Switch2/1
  Pos_Slope/1 -> Sum1/2
  Prev_Output/1 -> Sum/1, Sum1/1
  Neg_Slope/1 -> Sum/2

== system AEMS_Standard_Library/DISCONTINUITIES/AEMS_SLOPE_SWITCH_8INPUTS/Slope_On_Block/Error_Due_To_High_Slope_Test ==
  Signal_Change : Inport
  Output_Less_Than_Input : Inport  Port=2
  Output_Greater_Than_Input : Inport  Port=3
  Logical_Operator1 : Logic  Operator=OR  OutDataTypeStr=boolean
  Relational_Operator3 : RelationalOperator  Operator=~=  OutDataTypeStr=boolean  RndMeth=Nearest  InputSameDT=on
  Unit_Delay1 : UnitDelay  SampleTime=-1
      settings: AttributesFormatString=IC = %<X0>
  Test_passed : Outport
  wires:
  Logical_Operator1/1 -> Test_passed/1
  Signal_Change/1 -> Logical_Operator1/1
  Output_Less_Than_Input/1 -> Unit_Delay1/1
  Output_Greater_Than_Input/1 -> Relational_Operator3/1
  Relational_Operator3/1 -> Logical_Operator1/2
  Unit_Delay1/1 -> Relational_Operator3/2

== system AEMS_Standard_Library/DISCONTINUITIES/AEMS_SLOPE_SWITCH_8INPUTS/Slope_On_Block/Output_Comparision ==
  Test_passed : Inport
  Input : Inport  Tag=AM,In,0,1,Name,C;CMP,Port,PortWidth,SampleTime;  Port=2
  Pos_Slope : Inport  Tag=AM,In,0,1,Name,C;CMP,Port,PortWidth,SampleTime;  Port=3
  Prev_Output : Inport  Port=4
  Neg_Slope : Inport  Tag=AM,In,0,1,Name,C;CMP,Port,PortWidth,SampleTime;  Port=5
  LogicalOperator : Logic  Operator=OR  OutDataTypeStr=boolean
  Logical_Operator2 : Logic  OutDataTypeStr=boolean
  Relational_Operator1 : RelationalOperator  Operator=>  OutDataTypeStr=boolean  RndMeth=Nearest  InputSameDT=on
  Relational_Operator2 : RelationalOperator  Operator=<  OutDataTypeStr=boolean  RndMeth=Nearest  InputSameDT=on
  Sum : Sum  OutDataTypeStr=Inherit: Inherit via back propagation  RndMeth=Zero  SaturateOnIntegerOverflow=on  InputSameDT=on
      settings: AttributesFormatString=SAT = %<SaturateOnIntegerOverflow>
  Sum1 : Sum  OutDataTypeStr=Inherit: Inherit via back propagation  RndMeth=Zero  SaturateOnIntegerOverflow=on  InputSameDT=on
      settings: AttributesFormatString=SAT = %<SaturateOnIntegerOverflow>
  Switch1 : Switch  Tag=GEN,Threshold;AM,Switch,2,1;CMP,Threshold;  Criteria=u2 ~= 0  RndMeth=Zero  SaturateOnIntegerOverflow=on  InputSameDT=on
      settings: AttributesFormatString=Criteria=%<Criteria>
  Switch2 : Switch  Tag=GEN,Threshold;AM,Switch,2,1;CMP,Threshold;  Criteria=u2 ~= 0  RndMeth=Zero  SaturateOnIntegerOverflow=on  InputSameDT=on
      settings: AttributesFormatString=Criteria=%<Criteria>
  Switch3 : Switch  Tag=GEN,Threshold;AM,Switch,2,1;CMP,Threshold;  Criteria=u2 ~= 0  RndMeth=Zero  SaturateOnIntegerOverflow=on  InputSameDT=on
      settings: AttributesFormatString=Criteria=%<Criteria>
  Output_Not_Equals_Input : Outport  Tag=AM,Out,1,0,Name,NC;CMP,Port,OutputWhenDisabled,InitialOutput;
  Output : Outport  Tag=AM,Out,1,0,Name,NC;CMP,Port,OutputWhenDisabled,InitialOutput;  Port=2
  RelOp2_out : Outport  Tag=AM,Out,1,0,Name,NC;CMP,Port,OutputWhenDisabled,InitialOutput;  Port=3
  RelOp1_out : Outport  Tag=AM,Out,1,0,Name,NC;CMP,Port,OutputWhenDisabled,InitialOutput;  Port=4
  wires:
  Switch1/1 -> Switch2/3
  Relational_Operator2/1 -> RelOp2_out/1, LogicalOperator/1, Switch2/2
  Relational_Operator1/1 -> Switch1/2, LogicalOperator/2, RelOp1_out/1
  Sum/1 -> Relational_Operator1/1, Switch1/1
  Input/1 -> Relational_Operator2/2, Switch3/3, Relational_Operator1/2, Switch1/3
  Switch2/1 -> Switch3/1
  Logical_Operator2/1 -> Output_Not_Equals_Input/1
  LogicalOperator/1 -> Logical_Operator2/2
  Switch3/1 -> Output/1
  Test_passed/1 -> Switch3/2, Logical_Operator2/1
  Sum1/1 -> Relational_Operator2/1, Switch2/1
  Pos_Slope/1 -> Sum1/2
  Prev_Output/1 -> Sum/1, Sum1/1
  Neg_Slope/1 -> Sum/2

== system AEMS_Standard_Library/MATH/AEMS_IGN_TO_PHY/Inverse_order/Subsystem1 ==
  In : Inport
  Order_vector : Inport  Port=2
  Constant : Constant  OutDataTypeStr=Inherit: Inherit via back propagation
  Constant1 : Constant  Value=2  OutDataTypeStr=Inherit: Inherit via back propagation
  Constant2 : Constant  Value=3  OutDataTypeStr=Inherit: Inherit via back propagation
  Constant3 : Constant  Value=4  OutDataTypeStr=Inherit: Inherit via back propagation
  Constant4 : Constant  Value=5  OutDataTypeStr=Inherit: Inherit via back propagation
  Constant5 : Constant  Value=6  OutDataTypeStr=Inherit: Inherit via back propagation
  Constant6 : Constant  Value=0  OutDataTypeStr=Inherit: Inherit via back propagation
  Demux3 : Demux  Outputs=6
  RelationalOperator2 : RelationalOperator  Operator===  OutDataTypeStr=boolean  RndMeth=Nearest  InputSameDT=on
  Switch{,1..5} (6 alike) : Switch  Criteria=u2 ~= 0  RndMeth=Zero  SaturateOnIntegerOverflow=on  InputSameDT=on
      settings: AttributesFormatString=Criteria=%<Criteria>
  Out : Outport
  wires:
  RelationalOperator2/1 -> Demux3/1
  Demux3/1 -> Switch/2
  Demux3/2 -> Switch1/2
  Demux3/3 -> Switch2/2
  Demux3/4 -> Switch3/2
  Switch4/1 -> Switch3/3
  Demux3/5 -> Switch4/2
  Constant/1 -> Switch/1
  Constant1/1 -> Switch1/1
  Constant2/1 -> Switch2/1
  Constant3/1 -> Switch3/1
  Constant4/1 -> Switch4/1
  Switch3/1 -> Switch2/3
  Switch2/1 -> Switch1/3
  Switch1/1 -> Switch/3
  Order_vector/1 -> RelationalOperator2/2
  Switch/1 -> Out/1
  In/1 -> RelationalOperator2/1
  Demux3/6 -> Switch5/2
  Switch5/1 -> Switch4/3
  Constant5/1 -> Switch5/1
  Constant6/1 -> Switch5/3

== system AEMS_Standard_Library/MATH/AEMS_IGN_TO_PHY/Inverse_order/Subsystem2 ==
  In : Inport
  Order_vector : Inport  Port=2
  Constant : Constant  OutDataTypeStr=Inherit: Inherit via back propagation
  Constant1 : Constant  Value=2  OutDataTypeStr=Inherit: Inherit via back propagation
  Constant2 : Constant  Value=3  OutDataTypeStr=Inherit: Inherit via back propagation
  Constant3 : Constant  Value=4  OutDataTypeStr=Inherit: Inherit via back propagation
  Constant4 : Constant  Value=5  OutDataTypeStr=Inherit: Inherit via back propagation
  Constant5 : Constant  Value=6  OutDataTypeStr=Inherit: Inherit via back propagation
  Constant6 : Constant  Value=0  OutDataTypeStr=Inherit: Inherit via back propagation
  Demux3 : Demux  Outputs=6
  RelationalOperator2 : RelationalOperator  Operator===  OutDataTypeStr=boolean  RndMeth=Nearest  InputSameDT=on
  Switch{,1..5} (6 alike) : Switch  Criteria=u2 ~= 0  RndMeth=Zero  SaturateOnIntegerOverflow=on  InputSameDT=on
      settings: AttributesFormatString=Criteria=%<Criteria>
  Out : Outport
  wires:
  Constant6/1 -> Switch5/3
  Constant5/1 -> Switch5/1
  Switch5/1 -> Switch4/3
  Demux3/6 -> Switch5/2
  In/1 -> RelationalOperator2/1
  Switch/1 -> Out/1
  Order_vector/1 -> RelationalOperator2/2
  Switch1/1 -> Switch/3
  Switch2/1 -> Switch1/3
  Switch3/1 -> Switch2/3
  Constant4/1 -> Switch4/1
  Constant3/1 -> Switch3/1
  Constant2/1 -> Switch2/1
  Constant1/1 -> Switch1/1
  Constant/1 -> Switch/1
  Demux3/5 -> Switch4/2
  Switch4/1 -> Switch3/3
  Demux3/4 -> Switch3/2
  Demux3/3 -> Switch2/2
  Demux3/2 -> Switch1/2
  Demux3/1 -> Switch/2
  RelationalOperator2/1 -> Demux3/1

== system AEMS_Standard_Library/MATH/AEMS_IGN_TO_PHY/Inverse_order/Subsystem3 ==
  In : Inport
  Order_vector : Inport  Port=2
  Constant : Constant  OutDataTypeStr=Inherit: Inherit via back propagation
  Constant1 : Constant  Value=2  OutDataTypeStr=Inherit: Inherit via back propagation
  Constant2 : Constant  Value=3  OutDataTypeStr=Inherit: Inherit via back propagation
  Constant3 : Constant  Value=4  OutDataTypeStr=Inherit: Inherit via back propagation
  Constant4 : Constant  Value=5  OutDataTypeStr=Inherit: Inherit via back propagation
  Constant5 : Constant  Value=6  OutDataTypeStr=Inherit: Inherit via back propagation
  Constant6 : Constant  Value=0  OutDataTypeStr=Inherit: Inherit via back propagation
  Demux3 : Demux  Outputs=6
  RelationalOperator2 : RelationalOperator  Operator===  OutDataTypeStr=boolean  RndMeth=Nearest  InputSameDT=on
  Switch{,1..5} (6 alike) : Switch  Criteria=u2 ~= 0  RndMeth=Zero  SaturateOnIntegerOverflow=on  InputSameDT=on
      settings: AttributesFormatString=Criteria=%<Criteria>
  Out : Outport
  wires:
  RelationalOperator2/1 -> Demux3/1
  Demux3/1 -> Switch/2
  Demux3/2 -> Switch1/2
  Demux3/3 -> Switch2/2
  Demux3/4 -> Switch3/2
  Switch4/1 -> Switch3/3
  Demux3/5 -> Switch4/2
  Constant/1 -> Switch/1
  Constant1/1 -> Switch1/1
  Constant2/1 -> Switch2/1
  Constant3/1 -> Switch3/1
  Constant4/1 -> Switch4/1
  Switch3/1 -> Switch2/3
  Switch2/1 -> Switch1/3
  Switch1/1 -> Switch/3
  Order_vector/1 -> RelationalOperator2/2
  Switch/1 -> Out/1
  In/1 -> RelationalOperator2/1
  Demux3/6 -> Switch5/2
  Switch5/1 -> Switch4/3
  Constant5/1 -> Switch5/1
  Constant6/1 -> Switch5/3

== system AEMS_Standard_Library/MATH/AEMS_IGN_TO_PHY/Inverse_order/Subsystem4 ==
  In : Inport
  Order_vector : Inport  Port=2
  Constant : Constant  OutDataTypeStr=Inherit: Inherit via back propagation
  Constant1 : Constant  Value=2  OutDataTypeStr=Inherit: Inherit via back propagation
  Constant2 : Constant  Value=3  OutDataTypeStr=Inherit: Inherit via back propagation
  Constant3 : Constant  Value=4  OutDataTypeStr=Inherit: Inherit via back propagation
  Constant4 : Constant  Value=5  OutDataTypeStr=Inherit: Inherit via back propagation
  Constant5 : Constant  Value=6  OutDataTypeStr=Inherit: Inherit via back propagation
  Constant6 : Constant  Value=0  OutDataTypeStr=Inherit: Inherit via back propagation
  Demux3 : Demux  Outputs=6
  RelationalOperator2 : RelationalOperator  Operator===  OutDataTypeStr=boolean  RndMeth=Nearest  InputSameDT=on
  Switch{,1..5} (6 alike) : Switch  Criteria=u2 ~= 0  RndMeth=Zero  SaturateOnIntegerOverflow=on  InputSameDT=on
      settings: AttributesFormatString=Criteria=%<Criteria>
  Out : Outport
  wires:
  RelationalOperator2/1 -> Demux3/1
  Demux3/1 -> Switch/2
  Demux3/2 -> Switch1/2
  Demux3/3 -> Switch2/2
  Demux3/4 -> Switch3/2
  Switch4/1 -> Switch3/3
  Demux3/5 -> Switch4/2
  Constant/1 -> Switch/1
  Constant1/1 -> Switch1/1
  Constant2/1 -> Switch2/1
  Constant3/1 -> Switch3/1
  Constant4/1 -> Switch4/1
  Switch3/1 -> Switch2/3
  Switch2/1 -> Switch1/3
  Switch1/1 -> Switch/3
  Order_vector/1 -> RelationalOperator2/2
  Switch/1 -> Out/1
  In/1 -> RelationalOperator2/1
  Demux3/6 -> Switch5/2
  Switch5/1 -> Switch4/3
  Constant5/1 -> Switch5/1
  Constant6/1 -> Switch5/3

== system AEMS_Standard_Library/MATH/AEMS_IGN_TO_PHY/Inverse_order/Subsystem5 ==
  In : Inport
  Order_vector : Inport  Port=2
  Constant : Constant  OutDataTypeStr=Inherit: Inherit via back propagation
  Constant1 : Constant  Value=2  OutDataTypeStr=Inherit: Inherit via back propagation
  Constant2 : Constant  Value=3  OutDataTypeStr=Inherit: Inherit via back propagation
  Constant3 : Constant  Value=4  OutDataTypeStr=Inherit: Inherit via back propagation
  Constant4 : Constant  Value=5  OutDataTypeStr=Inherit: Inherit via back propagation
  Constant5 : Constant  Value=6  OutDataTypeStr=Inherit: Inherit via back propagation
  Constant6 : Constant  Value=0  OutDataTypeStr=Inherit: Inherit via back propagation
  Demux3 : Demux  Outputs=6
  RelationalOperator2 : RelationalOperator  Operator===  OutDataTypeStr=boolean  RndMeth=Nearest  InputSameDT=on
  Switch{,1..5} (6 alike) : Switch  Criteria=u2 ~= 0  RndMeth=Zero  SaturateOnIntegerOverflow=on  InputSameDT=on
      settings: AttributesFormatString=Criteria=%<Criteria>
  Out : Outport
  wires:
  RelationalOperator2/1 -> Demux3/1
  Demux3/1 -> Switch/2
  Demux3/2 -> Switch1/2
  Demux3/3 -> Switch2/2
  Demux3/4 -> Switch3/2
  Switch4/1 -> Switch3/3
  Demux3/5 -> Switch4/2
  Constant/1 -> Switch/1
  Constant1/1 -> Switch1/1
  Constant2/1 -> Switch2/1
  Constant3/1 -> Switch3/1
  Constant4/1 -> Switch4/1
  Switch3/1 -> Switch2/3
  Switch2/1 -> Switch1/3
  Switch1/1 -> Switch/3
  Order_vector/1 -> RelationalOperator2/2
  Switch/1 -> Out/1
  In/1 -> RelationalOperator2/1
  Demux3/6 -> Switch5/2
  Switch5/1 -> Switch4/3
  Constant5/1 -> Switch5/1
  Constant6/1 -> Switch5/3

== system AEMS_Standard_Library/MATH/AEMS_IGN_TO_PHY/Inverse_order/Subsystem6 ==
  In : Inport
  Order_vector : Inport  Port=2
  Constant : Constant  OutDataTypeStr=Inherit: Inherit via back propagation
  Constant1 : Constant  Value=2  OutDataTypeStr=Inherit: Inherit via back propagation
  Constant2 : Constant  Value=3  OutDataTypeStr=Inherit: Inherit via back propagation
  Constant3 : Constant  Value=4  OutDataTypeStr=Inherit: Inherit via back propagation
  Constant4 : Constant  Value=5  OutDataTypeStr=Inherit: Inherit via back propagation
  Constant5 : Constant  Value=6  OutDataTypeStr=Inherit: Inherit via back propagation
  Constant6 : Constant  Value=0  OutDataTypeStr=Inherit: Inherit via back propagation
  Demux3 : Demux  Outputs=6
  RelationalOperator2 : RelationalOperator  Operator===  OutDataTypeStr=boolean  RndMeth=Nearest  InputSameDT=on
  Switch{,1..5} (6 alike) : Switch  Criteria=u2 ~= 0  RndMeth=Zero  SaturateOnIntegerOverflow=on  InputSameDT=on
      settings: AttributesFormatString=Criteria=%<Criteria>
  Out : Outport
  wires:
  RelationalOperator2/1 -> Demux3/1
  Demux3/1 -> Switch/2
  Demux3/2 -> Switch1/2
  Demux3/3 -> Switch2/2
  Demux3/4 -> Switch3/2
  Switch4/1 -> Switch3/3
  Demux3/5 -> Switch4/2
  Constant/1 -> Switch/1
  Constant1/1 -> Switch1/1
  Constant2/1 -> Switch2/1
  Constant3/1 -> Switch3/1
  Constant4/1 -> Switch4/1
  Switch3/1 -> Switch2/3
  Switch2/1 -> Switch1/3
  Switch1/1 -> Switch/3
  Order_vector/1 -> RelationalOperator2/2
  Switch/1 -> Out/1
  In/1 -> RelationalOperator2/1
  Demux3/6 -> Switch5/2
  Switch5/1 -> Switch4/3
  Constant5/1 -> Switch5/1
  Constant6/1 -> Switch5/3

== system AEMS_Standard_Library/MATH/AEMS_SORT/For_loop_1/For_loop_2 ==
  Index_loop : Inport
  Vector_to_sort : Inport  Port=2
  Comparison : Subsystem
  For Iterator : ForIterator  IterationSource=external  IndexMode=Zero-based  IterationVariableDataType=int8
  If : If  IfExpression=u1 == 1
  Permutation_false : Subsystem  TreatAsAtomicUnit=on
  Permutation_true : Subsystem  TreatAsAtomicUnit=on
  Switch : Switch  Criteria=u2 ~= 0
      settings: AttributesFormatString=Criteria=%<Criteria>
  UnitDelay : UnitDelay  InitialCondition=zeros(1,N)  SampleTime=-1  StateName=unit
      settings: AttributesFormatString=<initial=%<InitialCondition>>
  Unit_delay_vector : Subsystem
  "Sorted_vector " : Outport
  wires:
  Index_loop/1 -> For Iterator/1
  For Iterator/1 -> Unit_delay_vector/3(Index_vector), Comparison/2(Index_vector), Permutation_true/4(High_index)
  Comparison/2(High_value_Out) -> Permutation_true/1(High_value)
  Comparison/3(Low_value_Out) -> Permutation_true/2(Low_value)
  Comparison/4(Low_index_Out) -> Permutation_true/3(Low_index)
  Comparison/1(Relational_Operator_Boolean) -> Switch/2, If/1
  If/1 -> Permutation_true/Action
  Switch/1 -> "Sorted_vector "/1, UnitDelay/1
  Unit_delay_vector/1(Vector_being_sorted) -> Permutation_true/5(Vector), Permutation_false/1(Vector), Comparison/1(Vector)
  If/2 -> Permutation_false/Action
  Permutation_true/1(Permuted_vector) -> Switch/1
  Permutation_false/1(Non_permuted_vector) -> Switch/3
  Vector_to_sort/1 -> Unit_delay_vector/2(Vector_to_sort)
  UnitDelay/1 -> Unit_delay_vector/1(Previous_vector)

== system AEMS_Standard_Library/SPECIFIC/AEMS_AIR_BALANCE/MWI_Mani_Charge_Mass_Air_EGR/EGRMANI_permission ==
  Constant : Constant  Value=Cbx_extegr
  Constant1 : Constant  Value=Cbx_lpegrsys
  Logical Operator : Logic  OutDataTypeStr=boolean
  Logical Operator1 : Logic  Operator=NOT  OutDataTypeStr=boolean
  egrmani_cal_ok : Outport
  wires:
  Logical Operator/1 -> egrmani_cal_ok/1  "egrmani_cal_ok"
  Logical Operator1/1 -> Logical Operator/2
  Constant/1 -> Logical Operator/1
  Constant1/1 -> Logical Operator1/1
